simulink model "PMSMcontrolbenchmark"  (R2024b)
settings: Solver=VariableStepAuto  StartTime=0.0  StopTime=4  RelTol=1e-3
model workspace (MAT data in the model file):
  CA = 2
  F = 0
  J = 0.002
  Ld = 0.0025
  Lq = 0.0025
  Ls = 0.005
  Rs = 0.34
  Tprofile = 0
  Vdc = 200
  Wmprofile = 0
  fsw = 10000
  phi = 0.022
  pn = 4
undefined symbols (not defined in the file or in its folder): bias_fc1, bias_fc2, bias_fc3, bias_fc4, sigbuilder_block, weights_fc1, weights_fc2, weights_fc3, weights_fc4
libraries: neural x25, slpidlib x5, simulink x4, spsDCVoltageSourceLib x1, spsPermanentMagnetSynchronousMachineLib x1, spsSeriesRLCBranchLib x1, spsUniversalBridgeLib x1, spsVoltageMeasurementLib x1, spsabctodq0Lib x1, spsdq0toabcLib x1, spspowerguiLib x1
(part 2 of 2)

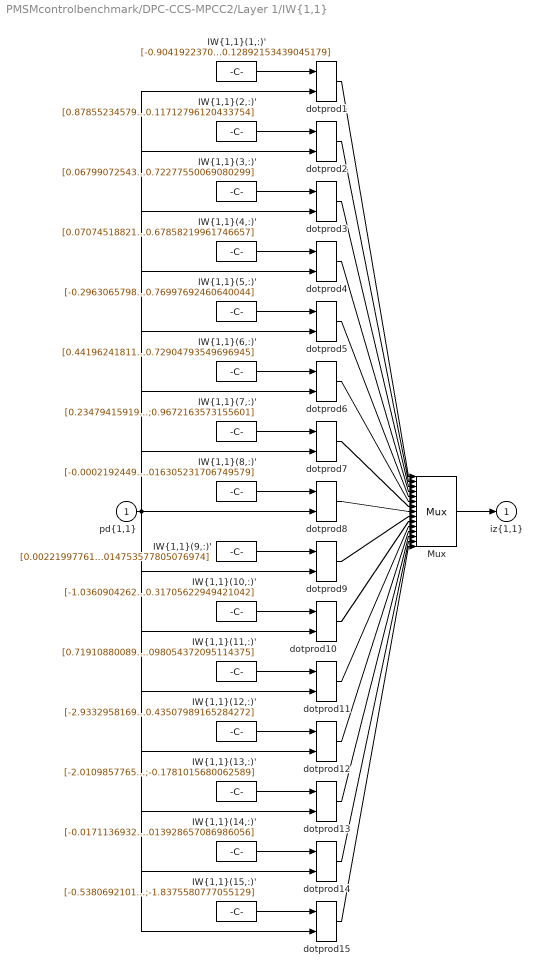
== system PMSMcontrolbenchmark/DPC-CCS-MPCC2/Layer 1/IW{1,1} ==
  "pd{1,1}" : Inport  PortDimensions=8
      mask Display: e = 0.06;c1 = [120 230 180]/255;c2 = ([120 230 180]+0)/(256+128);c3 = ([120 230 180]+128)/(256+128);patch([0 1 1 0],[0 0 1 1],c1);patch([0 1 1 1-e 1-e 0+e],[0 0 1 1-e 0+e 0+e],c2);patch([0 0 1 1-e 0+e 0+e],[0 1 1 1-e 1-e 0+e],c3);plot([0 1 1 0 0],[0 0 1 1 0]);
  "IW{1,1}(1,:)'" : Constant  Value=[-0.90419223707738372;-1.4343037631304167;0.84670863425173315;1.4592594100869951;0.10268997952413135;0.17192939610111693;-1.0947662886639049;-0.12892153439045179]
      mask Display: e = 0.06;c1 = [120 150 230]/255;c2 = ([120 150 230]+0)/383;c3 = ([120 150 230]+128)/383;patch([0 1 1 0],[0 0 1 1],c1);patch([0 1 1 1-e 1-e 0+e],[0 0 1 1-e 0+e 0+e],c2);patch([0 0 1 1-e 0+e 0+e],[0 1 1 1-e 1-e 0+e],c3);plot([0 1 1 0 0],[0 0 1 1 0]);disp('Weights');
  "IW{1,1}(10,:)'" : Constant  Value=[-1.0360904262833039;2.1269985950999963;1.0591578961575476;-1.8911947265654252;0.12222899356362021;-0.21454603214434087;1.0321689851653084;0.31705622949421042]
      mask Display: e = 0.06;c1 = [120 150 230]/255;c2 = ([120 150 230]+0)/383;c3 = ([120 150 230]+128)/383;patch([0 1 1 0],[0 0 1 1],c1);patch([0 1 1 1-e 1-e 0+e],[0 0 1 1-e 0+e 0+e],c2);patch([0 0 1 1-e 0+e 0+e],[0 1 1 1-e 1-e 0+e],c3);plot([0 1 1 0 0],[0 0 1 1 0]);disp('Weights');
  "IW{1,1}(11,:)'" : Constant  Value=[0.71910880089139229;-1.4954489577087631;-0.80577748632820378;1.3939860441659877;-0.094092007111237413;0.16232074219822765;-0.67261882429532494;0.098054372095114375]
      mask Display: e = 0.06;c1 = [120 150 230]/255;c2 = ([120 150 230]+0)/383;c3 = ([120 150 230]+128)/383;patch([0 1 1 0],[0 0 1 1],c1);patch([0 1 1 1-e 1-e 0+e],[0 0 1 1-e 0+e 0+e],c2);patch([0 0 1 1-e 0+e 0+e],[0 1 1 1-e 1-e 0+e],c3);plot([0 1 1 0 0],[0 0 1 1 0]);disp('Weights');
  "IW{1,1}(12,:)'" : Constant  Value=[-2.9332958169061718;0.24950066397585177;2.998994545044456;-0.027275261070770978;0.35933041538573646;-0.0012229000735380414;-0.56599808390398554;0.43507989165284272]
      mask Display: e = 0.06;c1 = [120 150 230]/255;c2 = ([120 150 230]+0)/383;c3 = ([120 150 230]+128)/383;patch([0 1 1 0],[0 0 1 1],c1);patch([0 1 1 1-e 1-e 0+e],[0 0 1 1-e 0+e 0+e],c2);patch([0 0 1 1-e 0+e 0+e],[0 1 1 1-e 1-e 0+e],c3);plot([0 1 1 0 0],[0 0 1 1 0]);disp('Weights');
  "IW{1,1}(13,:)'" : Constant  Value=[-2.0109857765623449;0.14703327323102056;1.9958868524356759;-0.010923897197350161;0.23355269112365887;-0.0017149046451916678;-0.4490699018195074;-0.1781015680062589]
      mask Display: e = 0.06;c1 = [120 150 230]/255;c2 = ([120 150 230]+0)/383;c3 = ([120 150 230]+128)/383;patch([0 1 1 0],[0 0 1 1],c1);patch([0 1 1 1-e 1-e 0+e],[0 0 1 1-e 0+e 0+e],c2);patch([0 0 1 1-e 0+e 0+e],[0 1 1 1-e 1-e 0+e],c3);plot([0 1 1 0 0],[0 0 1 1 0]);disp('Weights');
  "IW{1,1}(14,:)'" : Constant  Value=[-0.017113693211218018;-0.0047085532227480291;-0.012529267451761104;-0.0068990515421236513;0.0035053330091433447;-0.0017313021757524676;-10.112146048496369;-0.013928657086986056]
      mask Display: e = 0.06;c1 = [120 150 230]/255;c2 = ([120 150 230]+0)/383;c3 = ([120 150 230]+128)/383;patch([0 1 1 0],[0 0 1 1],c1);patch([0 1 1 1-e 1-e 0+e],[0 0 1 1-e 0+e 0+e],c2);patch([0 0 1 1-e 0+e 0+e],[0 1 1 1-e 1-e 0+e],c3);plot([0 1 1 0 0],[0 0 1 1 0]);disp('Weights');
  "IW{1,1}(15,:)'" : Constant  Value=[-0.53806921014410247;-0.92807915084975956;-0.75044570642532882;-0.74895352398937232;-0.13991626411514652;-0.11248354825213135;0.85478986648675137;-1.8375580777055129]
      mask Display: e = 0.06;c1 = [120 150 230]/255;c2 = ([120 150 230]+0)/383;c3 = ([120 150 230]+128)/383;patch([0 1 1 0],[0 0 1 1],c1);patch([0 1 1 1-e 1-e 0+e],[0 0 1 1-e 0+e 0+e],c2);patch([0 0 1 1-e 0+e 0+e],[0 1 1 1-e 1-e 0+e],c3);plot([0 1 1 0 0],[0 0 1 1 0]);disp('Weights');
  "IW{1,1}(2,:)'" : Constant  Value=[0.87855234579565511;1.4156624208614954;-0.80585990811740982;-1.4151503140528334;-0.096372498748147309;-0.16688634524379917;0.99960665147311112;-0.11712796120433754]
      mask Display: e = 0.06;c1 = [120 150 230]/255;c2 = ([120 150 230]+0)/383;c3 = ([120 150 230]+128)/383;patch([0 1 1 0],[0 0 1 1],c1);patch([0 1 1 1-e 1-e 0+e],[0 0 1 1-e 0+e 0+e],c2);patch([0 0 1 1-e 0+e 0+e],[0 1 1 1-e 1-e 0+e],c3);plot([0 1 1 0 0],[0 0 1 1 0]);disp('Weights');
  "IW{1,1}(3,:)'" : Constant  Value=[0.06799072543815686;0.17958946053952948;0.31087307044721013;0.50252571367343735;0.045283769407576502;0.080128130907266559;-0.25390057872751204;-0.72277550069080299]
      mask Display: e = 0.06;c1 = [120 150 230]/255;c2 = ([120 150 230]+0)/383;c3 = ([120 150 230]+128)/383;patch([0 1 1 0],[0 0 1 1],c1);patch([0 1 1 1-e 1-e 0+e],[0 0 1 1-e 0+e 0+e],c2);patch([0 0 1 1-e 0+e 0+e],[0 1 1 1-e 1-e 0+e],c3);plot([0 1 1 0 0],[0 0 1 1 0]);disp('Weights');
  "IW{1,1}(4,:)'" : Constant  Value=[0.070745188214225541;0.17961654516752218;0.60128249255245525;-0.84170941538096888;0.093952637532634359;-0.12359159785980574;0.3724369748825031;-0.67858219961746657]
      mask Display: e = 0.06;c1 = [120 150 230]/255;c2 = ([120 150 230]+0)/383;c3 = ([120 150 230]+128)/383;patch([0 1 1 0],[0 0 1 1],c1);patch([0 1 1 1-e 1-e 0+e],[0 0 1 1-e 0+e 0+e],c2);patch([0 0 1 1-e 0+e 0+e],[0 1 1 1-e 1-e 0+e],c3);plot([0 1 1 0 0],[0 0 1 1 0]);disp('Weights');
  "IW{1,1}(5,:)'" : Constant  Value=[-0.29630657986202363;0.19484317749671162;-0.48043924181345066;0.299590158569079;-0.075136768624160799;0.052281131266941644;-0.0550846972763534;-0.76997692460640044]
      mask Display: e = 0.06;c1 = [120 150 230]/255;c2 = ([120 150 230]+0)/383;c3 = ([120 150 230]+128)/383;patch([0 1 1 0],[0 0 1 1],c1);patch([0 1 1 1-e 1-e 0+e],[0 0 1 1-e 0+e 0+e],c2);patch([0 0 1 1-e 0+e 0+e],[0 1 1 1-e 1-e 0+e],c3);plot([0 1 1 0 0],[0 0 1 1 0]);disp('Weights');
  "IW{1,1}(6,:)'" : Constant  Value=[0.44196241811918469;-0.032055135187935603;-1.3142813844823593;0.11812388937772607;-0.17666452052034404;0.015896200837484057;0.17991657098907859;0.72904793549696945]
      mask Display: e = 0.06;c1 = [120 150 230]/255;c2 = ([120 150 230]+0)/383;c3 = ([120 150 230]+128)/383;patch([0 1 1 0],[0 0 1 1],c1);patch([0 1 1 1-e 1-e 0+e],[0 0 1 1-e 0+e 0+e],c2);patch([0 0 1 1-e 0+e 0+e],[0 1 1 1-e 1-e 0+e],c3);plot([0 1 1 0 0],[0 0 1 1 0]);disp('Weights');
  "IW{1,1}(7,:)'" : Constant  Value=[0.23479415919674354;0.31344263777582626;0.42059781507203292;0.37261119887377192;0.068073638845391873;0.061223043653048752;-0.32212857524313759;0.9672163573155601]
      mask Display: e = 0.06;c1 = [120 150 230]/255;c2 = ([120 150 230]+0)/383;c3 = ([120 150 230]+128)/383;patch([0 1 1 0],[0 0 1 1],c1);patch([0 1 1 1-e 1-e 0+e],[0 0 1 1-e 0+e 0+e],c2);patch([0 0 1 1-e 0+e 0+e],[0 1 1 1-e 1-e 0+e],c3);plot([0 1 1 0 0],[0 0 1 1 0]);disp('Weights');
  "IW{1,1}(8,:)'" : Constant  Value=[-0.00021924491660631359;0.015822682170862044;0.017853096757953411;-0.011932349049892016;0.0018407891691169069;-0.0030015758960702079;-10.860295797725927;0.016305231706749579]
      mask Display: e = 0.06;c1 = [120 150 230]/255;c2 = ([120 150 230]+0)/383;c3 = ([120 150 230]+128)/383;patch([0 1 1 0],[0 0 1 1],c1);patch([0 1 1 1-e 1-e 0+e],[0 0 1 1-e 0+e 0+e],c2);patch([0 0 1 1-e 0+e 0+e],[0 1 1 1-e 1-e 0+e],c3);plot([0 1 1 0 0],[0 0 1 1 0]);disp('Weights');
  "IW{1,1}(9,:)'" : Constant  Value=[0.0022199776122051296;0.02219272022769107;0.025672095869670113;0.010437498871763441;0.0071582324771227307;0.0023984309328512268;10.560252784389819;0.0014753577805076974]
      mask Display: e = 0.06;c1 = [120 150 230]/255;c2 = ([120 150 230]+0)/383;c3 = ([120 150 230]+128)/383;patch([0 1 1 0],[0 0 1 1],c1);patch([0 1 1 1-e 1-e 0+e],[0 0 1 1-e 0+e 0+e],c2);patch([0 0 1 1-e 0+e 0+e],[0 1 1 1-e 1-e 0+e],c3);plot([0 1 1 0 0],[0 0 1 1 0]);disp('Weights');
  Mux : Mux  Inputs=15
      mask Display: e = 0.06;c1 = [120 150 230]/255;c2 = ([120 150 230]+0)/383;c3 = ([120 150 230]+128)/383;patch([0 1 1 0],[0 0 1 1],c1);patch([0 1 1 1-e 1-e 0+e],[0 0 1 1-e 0+e 0+e],c2);patch([0 0 1 1-e 0+e 0+e],[0 1 1 1-e 1-e 0+e],c3);plot([0 1 1 0 0],[0 0 1 1 0]);disp('Mux');
  dotprod{1..15} (15 alike) : neural/Weight Functions/dotprod
  "iz{1,1}" : Outport
      mask Display: e = 0.06;c1 = [120 230 180]/255;c2 = ([120 230 180]+0)/(256+128);c3 = ([120 230 180]+128)/(256+128);patch([0 1 1 0],[0 0 1 1],c1);patch([0 1 1 1-e 1-e 0+e],[0 0 1 1-e 0+e 0+e],c2);patch([0 0 1 1-e 0+e 0+e],[0 1 1 1-e 1-e 0+e],c3);plot([0 1 1 0 0],[0 0 1 1 0]);
  wires:
  "IW{1,1}(1,:)'"/1 -> dotprod1/1
  "pd{1,1}"/1 -> dotprod1/2, dotprod2/2, dotprod3/2, dotprod4/2, dotprod5/2, dotprod6/2, dotprod7/2, dotprod8/2, dotprod9/2, dotprod10/2, dotprod11/2, dotprod12/2, dotprod13/2, dotprod14/2, dotprod15/2
  dotprod1/1 -> Mux/1
  "IW{1,1}(2,:)'"/1 -> dotprod2/1
  dotprod2/1 -> Mux/2
  "IW{1,1}(3,:)'"/1 -> dotprod3/1
  dotprod3/1 -> Mux/3
  "IW{1,1}(4,:)'"/1 -> dotprod4/1
  dotprod4/1 -> Mux/4
  "IW{1,1}(5,:)'"/1 -> dotprod5/1
  dotprod5/1 -> Mux/5
  "IW{1,1}(6,:)'"/1 -> dotprod6/1
  dotprod6/1 -> Mux/6
  "IW{1,1}(7,:)'"/1 -> dotprod7/1
  dotprod7/1 -> Mux/7
  "IW{1,1}(8,:)'"/1 -> dotprod8/1
  dotprod8/1 -> Mux/8
  "IW{1,1}(9,:)'"/1 -> dotprod9/1
  dotprod9/1 -> Mux/9
  "IW{1,1}(10,:)'"/1 -> dotprod10/1
  dotprod10/1 -> Mux/10
  "IW{1,1}(11,:)'"/1 -> dotprod11/1
  dotprod11/1 -> Mux/11
  "IW{1,1}(12,:)'"/1 -> dotprod12/1
  dotprod12/1 -> Mux/12
  "IW{1,1}(13,:)'"/1 -> dotprod13/1
  dotprod13/1 -> Mux/13
  "IW{1,1}(14,:)'"/1 -> dotprod14/1
  dotprod14/1 -> Mux/14
  "IW{1,1}(15,:)'"/1 -> dotprod15/1
  dotprod15/1 -> Mux/15
  Mux/1 -> "iz{1,1}"/1

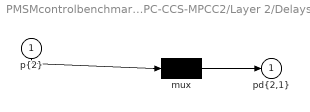
== system PMSMcontrolbenchmark/DPC-CCS-MPCC2/Layer 2/Delays 1 ==
  "p{2}" : Inport  PortDimensions=15
      mask Display: e = 0.06;c1 = [120 230 180]/255;c2 = ([120 230 180]+0)/(256+128);c3 = ([120 230 180]+128)/(256+128);patch([0 1 1 0],[0 0 1 1],c1);patch([0 1 1 1-e 1-e 0+e],[0 0 1 1-e 0+e 0+e],c2);patch([0 0 1 1-e 0+e 0+e],[0 1 1 1-e 1-e 0+e],c3);plot([0 1 1 0 0],[0 0 1 1 0]);
  mux : Mux  Inputs=1
      mask Display: e = 0.06;c1 = [120 150 230]/255;c2 = ([120 150 230]+0)/383;c3 = ([120 150 230]+128)/383;patch([0 1 1 0],[0 0 1 1],c1);patch([0 1 1 1-e 1-e 0+e],[0 0 1 1-e 0+e 0+e],c2);patch([0 0 1 1-e 0+e 0+e],[0 1 1 1-e 1-e 0+e],c3);plot([0 1 1 0 0],[0 0 1 1 0]);disp('Mux')
  "pd{2,1}" : Outport
      mask Display: e = 0.06;c1 = [120 230 180]/255;c2 = ([120 230 180]+0)/(256+128);c3 = ([120 230 180]+128)/(256+128);patch([0 1 1 0],[0 0 1 1],c1);patch([0 1 1 1-e 1-e 0+e],[0 0 1 1-e 0+e 0+e],c2);patch([0 0 1 1-e 0+e 0+e],[0 1 1 1-e 1-e 0+e],c3);plot([0 1 1 0 0],[0 0 1 1 0]);
  wires:
  "p{2}"/1 -> mux/1
  mux/1 -> "pd{2,1}"/1

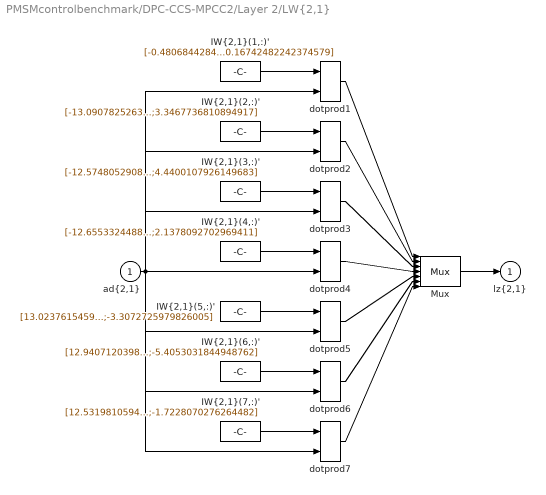
== system PMSMcontrolbenchmark/DPC-CCS-MPCC2/Layer 2/LW{2,1} ==
  "ad{2,1}" : Inport  PortDimensions=15
      mask Display: e = 0.06;c1 = [120 230 180]/255;c2 = ([120 230 180]+0)/(256+128);c3 = ([120 230 180]+128)/(256+128);patch([0 1 1 0],[0 0 1 1],c1);patch([0 1 1 1-e 1-e 0+e],[0 0 1 1-e 0+e 0+e],c2);patch([0 0 1 1-e 0+e 0+e],[0 1 1 1-e 1-e 0+e],c3);plot([0 1 1 0 0],[0 0 1 1 0]);
  "IW{2,1}(1,:)'" : Constant  Value=[-0.48068442845566089;-0.77896586602832385;0.054234845377817822;-0.51975255698429612;0.34660648033353519;0.19727111769818692;0.28300426105949794;-0.28729327339732824;-0.07108799595046851;-0.20073876991057454;-0.018441210928147735;0.017176020465646112;-0.23332259581077733;0.028855681088329296;0.16742482242374579]
      mask Display: e = 0.06;c1 = [120 150 230]/255;c2 = ([120 150 230]+0)/383;c3 = ([120 150 230]+128)/383;patch([0 1 1 0],[0 0 1 1],c1);patch([0 1 1 1-e 1-e 0+e],[0 0 1 1-e 0+e 0+e],c2);patch([0 0 1 1-e 0+e 0+e],[0 1 1 1-e 1-e 0+e],c3);plot([0 1 1 0 0],[0 0 1 1 0]);disp('weights');
  "IW{2,1}(2,:)'" : Constant  Value=[-13.090782526377641;11.758485673427447;-7.7027172426051038;-6.7398661562092572;12.199313640321435;11.060220205255234;-8.3706073098709872;-11.155216998960436;-13.246008856084668;-7.674193221427819;11.555148330510777;-7.4738470699062827;-9.477587005726992;13.900313060743342;3.3467736810894917]
      mask Display: e = 0.06;c1 = [120 150 230]/255;c2 = ([120 150 230]+0)/383;c3 = ([120 150 230]+128)/383;patch([0 1 1 0],[0 0 1 1],c1);patch([0 1 1 1-e 1-e 0+e],[0 0 1 1-e 0+e 0+e],c2);patch([0 0 1 1-e 0+e 0+e],[0 1 1 1-e 1-e 0+e],c3);plot([0 1 1 0 0],[0 0 1 1 0]);disp('weights');
  "IW{2,1}(3,:)'" : Constant  Value=[-12.574805290840933;11.701056154120211;-14.949859519831817;8.7419880664366882;-2.3079448995205665;9.8348747946801716;-13.237074031925085;5.2605750655565782;-12.881746685680186;8.0651492644250631;-13.037408185649793;-7.4031453882813558;-10.745565324774336;16.10535003688214;4.4400107926149683]
      mask Display: e = 0.06;c1 = [120 150 230]/255;c2 = ([120 150 230]+0)/383;c3 = ([120 150 230]+128)/383;patch([0 1 1 0],[0 0 1 1],c1);patch([0 1 1 1-e 1-e 0+e],[0 0 1 1-e 0+e 0+e],c2);patch([0 0 1 1-e 0+e 0+e],[0 1 1 1-e 1-e 0+e],c3);plot([0 1 1 0 0],[0 0 1 1 0]);disp('weights');
  "IW{2,1}(4,:)'" : Constant  Value=[-12.655332448851839;11.886241276869194;-10.007057663352805;9.5438320054961245;-15.066339203853822;-9.0251675203608279;-4.0621395957796134;16.870338026504367;2.1004102802706646;7.8064720158645553;-12.197836142702275;7.436606172184498;9.9547920023598682;1.2103825333930327;2.1378092702969411]
      mask Display: e = 0.06;c1 = [120 150 230]/255;c2 = ([120 150 230]+0)/383;c3 = ([120 150 230]+128)/383;patch([0 1 1 0],[0 0 1 1],c1);patch([0 1 1 1-e 1-e 0+e],[0 0 1 1-e 0+e 0+e],c2);patch([0 0 1 1-e 0+e 0+e],[0 1 1 1-e 1-e 0+e],c3);plot([0 1 1 0 0],[0 0 1 1 0]);disp('weights');
  "IW{2,1}(5,:)'" : Constant  Value=[13.023761545936793;-13.074755036794572;8.4024680079055383;6.4962652976628856;-12.207613385667315;-10.184961968307588;8.8621333976334302;10.479925940931661;13.280341406333124;7.0918895017185211;-12.272437483690966;7.2040614554183398;10.232889193801409;-13.739661561342603;-3.3072725979826005]
      mask Display: e = 0.06;c1 = [120 150 230]/255;c2 = ([120 150 230]+0)/383;c3 = ([120 150 230]+128)/383;patch([0 1 1 0],[0 0 1 1],c1);patch([0 1 1 1-e 1-e 0+e],[0 0 1 1-e 0+e 0+e],c2);patch([0 0 1 1-e 0+e 0+e],[0 1 1 1-e 1-e 0+e],c3);plot([0 1 1 0 0],[0 0 1 1 0]);disp('weights');
  "IW{2,1}(6,:)'" : Constant  Value=[12.940712039821419;-12.278757448139016;14.877192439108246;-9.248138366574354;2.4592715855591316;-9.6783751632331576;13.051417879204624;-5.8274426608852661;12.835483936315889;-8.3563998043042016;12.201599889995984;7.0838171303148796;10.478787962605068;-15.979816863163157;-5.4053031844948762]
      mask Display: e = 0.06;c1 = [120 150 230]/255;c2 = ([120 150 230]+0)/383;c3 = ([120 150 230]+128)/383;patch([0 1 1 0],[0 0 1 1],c1);patch([0 1 1 1-e 1-e 0+e],[0 0 1 1-e 0+e 0+e],c2);patch([0 0 1 1-e 0+e 0+e],[0 1 1 1-e 1-e 0+e],c3);plot([0 1 1 0 0],[0 0 1 1 0]);disp('weights');
  "IW{2,1}(7,:)'" : Constant  Value=[12.531981059481762;-12.820646080435997;10.460799203701455;-9.4449323590818199;15.355487277606741;9.7772670328941658;4.739445206144711;-17.464164600976304;-2.1818929035993331;-7.6249191088821044;12.155063181559283;-7.1741158819575155;-9.6214011692414623;-0.97617963352837422;-1.7228070276264482]
      mask Display: e = 0.06;c1 = [120 150 230]/255;c2 = ([120 150 230]+0)/383;c3 = ([120 150 230]+128)/383;patch([0 1 1 0],[0 0 1 1],c1);patch([0 1 1 1-e 1-e 0+e],[0 0 1 1-e 0+e 0+e],c2);patch([0 0 1 1-e 0+e 0+e],[0 1 1 1-e 1-e 0+e],c3);plot([0 1 1 0 0],[0 0 1 1 0]);disp('weights');
  Mux : Mux  Inputs=7
      mask Display: e = 0.06;c1 = [120 150 230]/255;c2 = ([120 150 230]+0)/383;c3 = ([120 150 230]+128)/383;patch([0 1 1 0],[0 0 1 1],c1);patch([0 1 1 1-e 1-e 0+e],[0 0 1 1-e 0+e 0+e],c2);patch([0 0 1 1-e 0+e 0+e],[0 1 1 1-e 1-e 0+e],c3);plot([0 1 1 0 0],[0 0 1 1 0]);disp('Mux');
  dotprod{1..7} (7 alike) : neural/Weight Functions/dotprod
  "lz{2,1}" : Outport
      mask Display: e = 0.06;c1 = [120 230 180]/255;c2 = ([120 230 180]+0)/(256+128);c3 = ([120 230 180]+128)/(256+128);patch([0 1 1 0],[0 0 1 1],c1);patch([0 1 1 1-e 1-e 0+e],[0 0 1 1-e 0+e 0+e],c2);patch([0 0 1 1-e 0+e 0+e],[0 1 1 1-e 1-e 0+e],c3);plot([0 1 1 0 0],[0 0 1 1 0]);
  wires:
  "IW{2,1}(1,:)'"/1 -> dotprod1/1
  "ad{2,1}"/1 -> dotprod1/2, dotprod2/2, dotprod3/2, dotprod4/2, dotprod5/2, dotprod6/2, dotprod7/2
  dotprod1/1 -> Mux/1
  "IW{2,1}(2,:)'"/1 -> dotprod2/1
  dotprod2/1 -> Mux/2
  "IW{2,1}(3,:)'"/1 -> dotprod3/1
  dotprod3/1 -> Mux/3
  "IW{2,1}(4,:)'"/1 -> dotprod4/1
  dotprod4/1 -> Mux/4
  "IW{2,1}(5,:)'"/1 -> dotprod5/1
  dotprod5/1 -> Mux/5
  "IW{2,1}(6,:)'"/1 -> dotprod6/1
  dotprod6/1 -> Mux/6
  "IW{2,1}(7,:)'"/1 -> dotprod7/1
  dotprod7/1 -> Mux/7
  Mux/1 -> "lz{2,1}"/1

== matlab function PMSMcontrolbenchmark/DPC-CCS-MPCC2/HiddenLayer4_ReLU1 ==
  data: u input; y output
function y = fcn(u)
% ReLU 激活函数
y = max(0, u);

== matlab function PMSMcontrolbenchmark/MATLAB Function4 ==
  data: id input size=[1,1]; u_opt output size=[1,2]; iq input size=[1,1]; iq_ref input size=[1,1]; omega_e input size=[1,1]; uoptold input; data_out output; outputs output
function [u_opt,data_out,outputs]  = pmsm_ccs_mpc(id, iq, iq_ref, omega_e,uoptold)
% PMSM CCS-MPC: compute optimal vd, vq for dq current tracking
% x(k+1) = A(omega_e)*x(k) + B*u(k) + c(omega_e)
%
% Inputs
%   id, iq      : measured currents in dq (A)
%   iq_ref      : outer-loop reference for iq (A). id_ref = 0 inside.
%   omega_e     : electrical angular speed (rad/s)
%   params      : struct with fields
%       Ts      : sampling time (s)
%       Rs      : stator resistance (ohm)
%       Ld, Lq  : dq-axis inductances (H)
%       psi_f   : PM flux (Wb)
%       N       : prediction horizon (default 3~5)
%       Qd, Qq  : current-tracking weights (default 1)
%       Rv_d, Rv_q : voltage weights (default small, e.g., 1e-4)
%       Vmax    : optional voltage limit for saturation (line-to-neutral, dq)
%
% Outputs
%   u_opt = [vd, vq]   : optimal dq voltages at k (apply via SVPWM)
%   dbg  : struct for debugging/prediction preview

% -------- parameters ----------


Ts   = 100e-6;
Rs   = 0.34;
Ld   = 2.5e-3;
Lq   = 2.5e-3;
psi_f= 0.022;
N    = 5;          % 预测域
Qd   = 5;          % |id-0|权重
Qq   = 5;          % |iq-iqref|权重
Rv_d = 0;       % 电压惩罚
Rv_q = 0;

% 
% Rs = 1.2;
% Ld = 0.0075;
% Lq = 0.0075;
% psi_f = 0.044;
% use_sat = isfield(params,'Vmax');
% if use_sat, Vmax = params.Vmax; end

% -------- linearized discrete model (Forward Euler) ----------
% id(k+1) = id + Ts/Ld*(vd - Rs*id + w_e*Lq*iq)
% iq(k+1) = iq + Ts/Lq*(vq - Rs*iq - w_e*(Ld*id + psi_f))

% A = [ 1 - Ts*Rs/Ld,   Ts*omega_e*Lq/Ld; ...
%      -Ts*omega_e*Ld/Lq, 1 - Ts*Rs/Lq ];
% 
% B = [ Ts/Ld,  0; ...
%       0,     Ts/Lq ];
% 
% c = [ 0;  -Ts*omega_e*psi_f/Lq ];


Ac = [-Rs/Ld,          omega_e*Lq/Ld;
      -omega_e*Ld/Lq, -Rs/Lq];
Bc = [1/Ld, 0;
      0,    1/Lq];
dc = [0; -omega_e*psi_f/Lq];

I  = eye(2);
M  = (I - 0.5*Ts*Ac);          % must be invertible (常规参数下成立)

A = M \ (I + 0.5*Ts*Ac);      % (I - Ts/2 Ac)^(-1) (I + Ts/2 Ac)
B = M \ (Ts * Bc);            % (I - Ts/2 Ac)^(-1) Ts Bc
c = M \ (Ts * dc);            % (I - Ts/2 Ac)^(-1) Ts dc

% -------- build stacked prediction: X = Phi*x0 + Gamma*U + D ----------
x0 = [id; iq];
% x0 = A*x0 + B*uoptold(:) + c; 

% weights
Q = diag([Qd, Qq]);
R = blkdiag(kron(eye(N), diag([Rv_d, Rv_q])));   % 2N x 2N
Qblk = kron(eye(N), Q);                           % 2N x 2N

% Pre-compute powers of A
Phi = [];
Gamma = [];
D = [];
Ai = eye(2);
d_i = [0;0];

for i = 1:N
    Ai = A*Ai;                      % A^i (note: Ai holds A^i at end of loop)
    Phi = [Phi; Ai];

    % build Gamma row block  [A^(i-1)B  A^(i-2)B ... B  0 ... 0]
    Gi = [];
    for j = 1:i
        Gi = [Gi, A^(i-j)*B];
    end
    Gi = [Gi, zeros(2, 2*(N-i))];   % pad to 2 x (2N)
    Gamma = [Gamma; Gi];

    % affine term sum_{j=0}^{i-1} A^{i-1-j} * c
    d_i = A^(i-1)*c + d_i;          % iterative sum
    D = [D; d_i];
end

% Reference stack: [0; iq_ref] repeated
xref = repmat([0; iq_ref], N, 1);

% -------- convex QP in closed form (unconstrained) ----------
% J = || (Phi*x0 + Gamma*U + D) - xref ||_Qblk^2 + U^T R U
% -> H = Gamma' Qblk Gamma + R ;  f = 2 Gamma' Qblk (Phi*x0 + D - xref)
E = Phi*x0 + D - xref;
H = Gamma.' * Qblk * Gamma + R;
% f = 2 * (E.' * Qblk * Gamma).';
% f = 2 * ( Gamma.' * Qblk * E  -  R * uoptold(:) );  % 
f = 2 * ( Gamma.' * Qblk * E);  % 

% small regularization for numerical safety
% H = H + 1e-10*eye(size(H));


Uopt = -0.5 * (H \ f);   % 2N x 1   [vd(k); vq(k); vd(k+1); ...]
vd = Uopt(1);
vq = Uopt(2);

% optional voltage saturation (dq circle)
% if use_sat
%     Vnorm = hypot(vd, vq);
%     if Vnorm > Vmax
%         scale = Vmax / Vnorm;
%         vd = vd*scale; vq = vq*scale;
%     end
% end

u_opt = [vd, vq];
data_out=[id, iq, iq_ref, omega_e];

% % -------- debug info --------
% % predict first-step state with chosen u_opt
% x1 = A*x0 + B*u_opt.' + c;
% dbg.A = A; dbg.B = B; dbg.c = c;
% dbg.Phi = Phi; dbg.Gamma = Gamma; dbg.D = D;
% dbg.x0 = x0; dbg.xref = xref; dbg.Uopt = Uopt;
% dbg.x1 = x1; dbg.cost = (E + Gamma*Uopt).' * Qblk * (E + Gamma*Uopt) + Uopt.'*R*Uopt;
bias_fc1=[0.45077223;-0.98593277;0;0.77458781;-0.044927038;-1.2634193;-1.1666412;1.7427140;1.1461650;-0.66138917;0;0.90436518;1.0436105;-0.67685294;0;1.1854513];
bias_fc2=[-0.089997061;-0.73082793;0.49555737;0.31255305;0.55459338;0.35870293;-1.0354316;1.1187282;0;-0.15719745;-0.96471405;0.27960911;-1.6519834;-0.68177450;-0.87690234;-1.7175794];
bias_fc3=[0.93791717;0.28083891;1.2938812;0.23406027;1.2630615;0.18311015;0.94357389;0.15088876;1.0176181;-0.018218765];

weights_fc1=[2.9836543,0.21754484,0.23341990,-0.26597860;-1.7504053,-0.071081415,0.33457848,0.30706480;-0.13166997,-0.47914264,-0.45795056,-0.43386942;-2.3850040,-0.38283822,-0.29051980,0.37873942;-1.9668556,0.37444186,0.13269018,-0.53277105;2.1087008,-0.026306434,0.50306749,0.16578338;-0.34209993,0.21763547,0.51496810,0.32770357;-0.87144250,-0.33639261,-0.046674166,0.019663444;-0.30909187,-0.36187267,-0.51643550,0.082297631;1.6132237,0.018911676,0.15870258,0.49692670;0.24044013,-0.49206474,-0.11636607,-0.21767166;-2.2360814,0.084858932,-0.52798504,0.50181317;1.4347870,-0.45848849,-0.068210639,0.53975832;2.4921572,-0.066860348,0.20898369,0.37398779;-0.22073913,-0.44315240,-0.44243282,-0.039189480;0.79985756,0.26092672,-0.62605429,0.30781415];
weights_fc2=[-0.28554773,0.24336202,-0.25427419,-0.41032195,-0.39795434,0.23006199,-0.013505463,-0.28364414,0.093326397,-0.51943278,-0.37646031,-0.48641306,-0.11188874,0.24040596,0.36509323,-0.35647205;0.48697984,0.26366106,0.21134749,-0.27952978,0.048428819,-0.12448037,0.39424112,-0.56977713,-0.18103860,0.35486746,0.42267683,-0.052898254,-0.18843828,0.040900275,-0.24224217,-0.12835120;0.23481733,-0.46081695,0.11310379,0.33427963,-0.055886380,-0.13837937,0.022537103,0.47408611,0.36451611,0.29569119,-0.18022014,0.063691236,-0.22106594,0.15140918,0.26968431,0.34181863;0.10248613,0.41877151,0.20655465,-0.18769953,-0.27901343,0.34030330,0.55757183,-0.071869865,-1.0280613,-0.32102242,0.32338384,0.30249843,-0.35028249,-0.27652812,0.42958483,-0.029763365;-0.20040011,0.22723116,0.21474153,0.033300426,-0.32844585,-0.38157380,-0.11579093,0.24342629,0.13367273,0.26715124,-0.41963884,-0.30545336,0.39054000,-0.035623550,-0.16873537,-0.34092751;-0.33662999,-0.16656519,-0.29985607,-0.095112823,0.45188391,0.39926216,0.55219311,0.076473899,-0.58229911,0.098838329,0.31828493,-0.30524421,-0.10214633,0.12343165,-0.11838164,-0.27259079;-0.25555626,0.36243561,-0.052402027,0.13044976,0.44660312,0.13083866,0.31027490,-0.82364202,0.34670842,-0.021939194,-0.26410505,-0.12682776,-0.31633902,0.20819357,-0.10657405,0.33853766;-0.40919405,-0.32170519,-0.21678893,0.069650635,-0.33320588,-0.29535475,-0.27024373,0.84402943,0.29002970,0.089938045,0.21562091,0.33956856,0.046714630,0.094360784,0.25361419,-0.046129491;0.42811784,-0.39747807,-0.070922568,0.28011781,-0.20151779,-0.24338481,-0.18568891,-0.15647404,0.065355800,0.28132591,-0.41860786,-0.24202845,-0.24852444,0.28573295,-0.27408409,0.10478047;0.88460881,-0.047915816,-0.12782235,-0.26589879,-0.019808091,-0.31095701,-0.032223962,-0.10295556,0.19449581,-0.030397819,-0.090301469,-0.094766393,0.36906600,0.29811588,-0.038152516,0.43641442;-0.21999909,0.36879671,0.30716559,0.12600207,0.19337425,-0.10735262,0.050037641,-0.51286554,0.20538558,-0.26924625,0.21295474,0.20841700,-0.31597853,0.33462280,-0.12048907,0.052154209;0.61092913,0.48729083,0.29494962,-0.29483396,0.029483441,-0.32239917,0.014563133,0.17354123,0.16326545,0.29814705,0.41145143,0.13658403,0.14763220,0.012346282,-0.051424358,-0.25855792;0.026253963,0.0041296668,-0.12525518,-0.27092993,0.23845407,0.17713882,-0.081141047,-1.7330632,-0.10933389,0.43198079,-0.39299470,-0.063535087,-0.27358279,0.26215911,-0.36818984,-0.14806621;0.14697802,-0.28067791,-0.045846056,-0.11016481,0.71082461,0.20501535,0.38714385,-0.072625108,0.22445719,0.46867910,-0.084716916,-0.10520785,-0.29460549,0.35037595,-0.036845554,-0.24545509;-0.33511752,-0.48108593,-0.017082207,0.044664353,0.23209597,0.16915733,0.078579046,0.63127023,0.74429131,-0.35985848,-0.14038230,0.012219186,0.36597079,-0.095396318,-0.16881314,0.26844075;0.56203765,-0.0089203632,0.33196288,-0.34847358,-0.46404761,0.56125927,0.20313917,-2.6953599,-0.89338851,-0.090183266,0.25846690,-0.058696277,0.33669561,-0.19577506,0.27903962,-0.11533026];
weights_fc3=[-0.36097988,-0.079362221,-0.050739940,1.0226167,-0.0035440219,0.56462848,0.27425730,-0.087315388,0.033870876,-0.15360855,-0.051583439,-0.093072563,-1.3137652,-0.11517673,-0.16721556,-1.5774437;-0.28031033,0.033889450,-0.24691170,0.12988298,-0.30705434,0.029123802,0.25188887,0.015227616,-0.085394859,0.18498293,0.027248941,-0.29693484,-0.45173821,0.42610627,0.094816618,-0.033691645;0.11722923,-0.15767683,0.20172533,0.63249391,0.064739250,0.55467516,-0.20113622,0.72799897,0.25163153,-0.27735814,-0.10170000,0.21215706,-1.2549610,-0.16126682,-0.71125031,-0.37614501;-0.0015062199,0.54359436,-0.17181879,0.14887026,-0.11275439,-0.032249484,-0.23578040,0.44388297,-0.30703741,0.48458320,0.37011936,-0.38601127,0.33312708,0.00037542792,-0.24785377,-0.058023591;-0.021428399,-0.36394218,0.49350199,1.1519299,0.65712833,0.53128660,-0.15991975,0.29033753,-0.034774959,0.40692419,-0.38373220,-0.35072601,-0.55021596,-0.36156699,-1.0848695,-0.65512282;-0.013191225,0.35796583,0.079549506,-0.30845693,-0.23991026,0.54874516,-0.31901610,0.025404388,-0.22365196,0.27552736,-0.38096401,0.30835944,-0.036030628,-0.091264449,-0.23291565,0.040350094;0.16536474,-0.31835166,-0.13170175,0.58550209,0.49252480,0.92714846,-0.43181959,0.077736624,0.34689656,-0.17002237,0.28111348,0.51249397,-1.2118325,-0.011065885,-0.54054403,-1.1135581;-0.091544293,0.18975821,-0.12975927,0.079746544,-0.30504933,-0.15370435,-0.36537498,0.46268797,-0.19949818,0.48752698,-0.33017454,0.17795384,0.40321833,0.13899876,-0.32418919,0.31619111;-0.24607334,-0.53155792,0.46883988,0.78695017,0.14787959,0.53385520,0.099893041,-0.077855349,-0.45045540,-0.39248264,-0.21902253,-0.067012377,-0.53684765,0.18791474,-0.42473134,-1.2862216;-0.38009945,0.55439764,-0.37049609,0.048198853,-0.029421648,-0.15018409,-0.16371690,-0.15938444,-0.38038316,-0.39580646,-0.33843836,0.67853087,-0.41232979,0.34779015,0.45513850,-0.54214072];





%%
% bias_fc1=[-0.21772923;0.081826821;0.060489286;0.052606367;0.18588531;0;0.016658101;0.051218331;-0.23023616;-0.30166718;0.31534657;0;-0.21972460;0.15919764;-0.0099884365;0.32744771];
% bias_fc2=[-0.064750440;-0.26559365;0.26059553;0;0.27747932;-0.10923114;-0.024771458;0.27032962;0;-0.29978201;-0.081293471;-0.12819004;-0.24896750;-0.0024433834;0;0.0031462451];
% bias_fc3=[0.16386688;0.053151917;0.25407600;0.23018189;0.24445285;-0.029745348;0.25700310;-0.040530961;0.11396128;-0.032071784];
% 
% weights_fc1=[0.24764431,-0.14868990,0.36363265,0.47946697;0.25133237,0.48908710,0.15724072,-0.35253334;-0.43726680,0.27101740,0.21058813,-0.21320398;0.019298214,0.43632972,-0.048476502,-0.28392375;0.12154109,-0.59161764,-0.18045776,0.43736523;0.16485953,-0.42591086,0.045330822,-0.51319355;0.28601292,0.50915271,0.26901904,-0.050234500;0.80911314,0.22678807,0.16371737,-0.30859870;0.0057375031,0.62647736,0.30853111,0.070813864;-0.16610269,-0.26449057,0.44193602,0.43936267;0.068810634,-0.70247120,-0.34436947,0.068125248;0.070045836,0.056100018,-0.50674623,-0.37554589;-0.047524836,0.52820539,0.41414836,0.27225837;0.26849180,0.087001875,-0.068890728,0.46406829;0.43422475,-0.49390489,0.50367582,-0.13475934;-0.79639244,-0.58797216,-0.013162494,0.32241136];
% weights_fc2=[0.079308510,-0.055751558,-0.31491882,-0.30550155,-0.40163979,-0.24682771,-0.069445558,0.25527209,0.25871587,0.33401388,-0.016689448,0.15235402,-0.35537058,-0.31268650,-0.24075900,-0.26408741;-0.011472629,0.24143729,-0.12036573,0.016271522,-0.32142583,0.37287018,-0.34229904,-0.19235387,-0.11705281,-0.11769364,-0.31403416,-0.0083105126,0.43322203,0.21736601,0.25487795,-0.097302765;-0.010481030,-0.081993453,0.28420925,0.013025627,-0.17161511,-0.23601627,0.31384975,0.010155731,-0.16855617,0.13956840,0.33217251,0.00012788722,0.42275140,0.21344049,-0.34047791,-0.36136308;-0.43030965,-0.11110848,0.32941636,-0.048444487,-0.14112432,0.12818350,0.19009195,-0.016897835,-0.24554458,0.19149487,-0.027648313,0.040777020,-0.045579817,-0.38339108,-0.11832730,0.092607021;-0.17528991,-0.43099299,-0.39926624,-0.18237565,0.12294805,0.061695769,-0.58868229,-0.37327173,-0.33396047,0.18290494,0.45844871,-0.40801021,-0.22611034,0.24512117,0.19973534,-0.13256167;-0.053971183,0.10997819,-0.34697673,-0.32642642,0.21448036,0.29142797,0.14517197,0.32793367,0.65686572,-0.042029180,-0.33355901,0.0024723869,0.34507313,-0.15629716,0.42900673,-0.070386760;-0.0080062468,-0.27809516,-0.10570976,0.013408719,0.22257613,0.041092522,0.17608121,0.43497252,0.34326354,-0.26400304,0.095730200,-0.33321857,0.39181882,-0.21485212,-0.20922475,-0.14390624;-0.054248549,0.079113841,0.16571839,-0.36497360,0.42255729,0.34934387,-0.0018455114,0.035704087,-0.40309232,-0.28277329,0.090932414,-0.30725262,-0.45150366,0.15950051,-0.36903691,0.42051935;-0.35759899,-0.31898952,0.089875154,0.35846439,0.011080389,-0.35085630,0.22275077,0.21751273,-0.16582726,-0.40838403,-0.22850287,0.33681113,-0.28020015,0.41559672,-0.42415872,0.0071374718;0.038228445,-0.083302729,-0.072092190,0.33026415,0.041646250,0.18022889,0.060295824,0.32073882,-0.014920481,0.35729596,-0.15305960,-0.059574611,-0.28132862,0.21448548,0.36382660,-0.33605102;-0.47060403,-0.37277830,-0.47946799,0.058652688,-0.25960565,-0.37767348,0.34199229,0.023822496,0.31589502,-0.31038848,-0.23949845,0.16992863,0.074903741,-0.48289832,0.26519457,0.31712094;0.32586810,0.086000986,0.12804388,0.34084257,-0.25940442,0.37749234,-0.14576210,0.052950095,-0.17219093,0.24590340,0.076417908,-0.048462756,0.11139538,-0.017329961,-0.17521530,-0.18081903;0.34698045,-0.032992747,0.13627613,-0.075201593,-0.0023707969,-0.36490285,-0.38291544,-0.053347282,-0.017152384,0.20760088,-0.12400562,-0.16071591,-0.21422029,-0.061265398,-0.37467197,-0.40086663;-0.43012351,0.13256823,-0.37590170,-0.095354453,-0.0031352248,-0.20722784,-0.24795784,0.37718847,-0.38331863,0.25138345,0.35932732,0.39169317,0.21417074,-0.21975341,-0.037654404,0.36432388;-0.24431077,0.26667163,-0.26484957,0.33212066,0.11778346,-0.18644144,-0.073916078,-0.16454287,-0.25540793,0.075874709,-0.020141367,0.13370328,0.17302415,-0.36253995,0.21435477,0.19951820;0.15023533,-0.12779802,0.21798261,0.31865078,0.24023996,0.30365649,0.027152516,-0.42147729,0.34220555,-0.12682286,-0.13084802,-0.14263426,-0.029751932,-0.14469312,0.26456028,-0.28339231];
% weights_fc3=[-0.16997327,-0.11862612,0.19308701,0.40131071,0.26927051,-0.57197672,0.21633384,0.11646987,0.20114695,-0.19254172,-0.25252065,0.070078738,-0.0041858144,-0.40196738,0.41337475,0.71409804;-0.19948561,0.18895768,-0.028998401,-0.41713709,-0.31463507,0.25712788,0.14127438,0.31889144,0.10877583,-0.48712534,0.095822230,0.40714744,0.10137367,0.23239236,-0.043016180,-0.25745106;0.47503909,-0.67516631,0.16558950,0.29054841,0.11431315,-0.018638812,0.17131688,0.21516931,0.32197735,0.012067144,-0.17478132,-0.52978361,-0.26175833,0.026900336,-0.46481812,-0.090804204;0.063100800,-0.29601094,0.40339646,0.016236722,-0.21809264,0.058128498,-0.0058182329,-0.017282460,0.34610030,-0.19409527,-0.065960124,0.14812869,-0.041373886,-0.034080375,-0.099996641,-0.091166347;-0.14358719,-0.032253630,0.47853890,-0.27436477,0.35874328,-0.33730048,-0.19635512,0.33269897,0.40211129,-0.44521213,-0.25620881,-0.059013944,-0.64009243,-0.057423402,-0.30281371,0.10445856;-0.38949299,0.037640464,-0.17367756,0.17898226,-0.080580182,0.43359783,0.063486643,0.15370663,-0.080662847,-0.22982912,-0.28774855,0.076002479,0.31372762,-0.38888046,0.46615428,0.16595097;0.43038404,-0.54802889,-0.15381087,-0.47789723,-0.035902318,-0.26002285,0.51511300,0.36825767,-0.22424302,-0.12464098,0.016186472,0.15703672,-0.44691542,0.37883586,0.42679185,0.12882048;-0.37625682,0.16615012,-0.13239466,0.14560121,-0.15972079,0.0091079306,0.14538717,-0.16719858,0.071672030,-0.13898522,0.019021524,0.64318639,-0.14770664,0.082423814,0.046032671,0.36352944;-0.42732984,0.090957642,-0.15953772,0.38931033,0.085008353,-0.14090097,0.34485719,0.52908450,-0.23254445,-0.35639673,0.30658177,-0.014483502,-0.024786673,0.26905370,-0.28459856,-0.045587737;-0.43085644,-0.073504932,0.40825680,-0.094283849,-0.31363520,0.19693558,-0.16355057,0.34359702,0.17143407,-0.22607051,-0.082455747,-0.17191108,0.31244513,0.34940949,-0.15200123,0.18822372];


output1=data_out*weights_fc1'+bias_fc1';
output1=max(0,output1);
output2=output1*weights_fc2'+bias_fc2';
output2=max(0,output2);
output=output2*weights_fc3'+bias_fc3';

outputs = output(:,1:2);


end

== matlab function PMSMcontrolbenchmark/DPC-CCS-MPCC2/HiddenLayer1_ReLU ==
  data: u input; y output
function y = fcn(u)
% ReLU 激活函数
y = max(0, u);

== matlab function PMSMcontrolbenchmark/DPC-CCS-MPCC2/HiddenLayer4_ReLU ==
  data: u input; y output
function y = fcn(u)
% ReLU 激活函数
y = max(0, u);

== matlab function PMSMcontrolbenchmark/DPC-CCS-MPCC2/HiddenLayer1_ReLU1 ==
  data: u input; y output
function y = fcn(u)
% ReLU 激活函数
y = max(0, u);

== matlab function PMSMcontrolbenchmark/DPC-CCS-MPCC2/HiddenLayer4_ReLU2 ==
  data: u input; y output
function y = fcn(u)
% ReLU 激活函数
y = max(0, u);
